simulink library "dspsigops"  (Simulink 8.2)
settings: Solver=ode45  SolverMode=SingleTasking  StartTime=0.0  StopTime=10.0  RelTol=1e-3
settings Model: RequirementInfo=9  ForwardingTableString=||__slOldName__||dspsigops/Zero Pad||__slNewName__||dspsigops/Pad||__slOldName__||dspsigops/Integer Delay||__slNewName__||dspobslib/Integer Delay  Creator=szlotkin  LastModifiedBy=mmclerno  CovMetricSettings=d  ExtModeAutoUpdateStatusClock=off

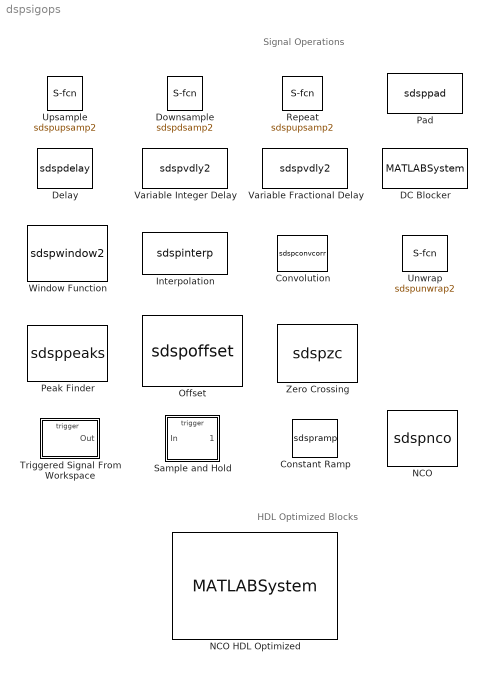
== system dspsigops ==
  note: Signal Operations
  note: HDL Optimized Blocks
  Constant Ramp : S-Function  FunctionName=sdspramp  Parameters=L, dim, Slope, Offset, isCustomFloat,isSigned,dTypeID,wordLength,fracBits,fracBitsMode  EnableBusSupport=off  mask(Constant Ramp){L=Rows, dim=1, Slope=1, Offset=0, additionalParams=off, allowOverrides=on, dataType=Same as input, isSigned=on, wordLen=16, udDataType=sfix(16), fracBitsMode=Best precision, numFracBits=15, OutDataTypeStr=Inherit: Same as input, LastOutDataTypeStr=Inherit: Same as input}
      mask prompts: L "Ramp length equals number of:"; dim "Dimension:"; additionalParams "------- Show additional parameters --------"; allowOverrides "Allow overrides from DSP Fixed-Point Attributes blocks"; dataType "Output data type:"; isSigned "Signed"; wordLen "Word length:"; udDataType "User-defined data type (e.g. sfix(16), float('single')):"; fracBitsMode "Set fraction length in output to:"; numFracBits "Fraction length:"; OutDataTypeStr "Output data type:"; LastOutDataTypeStr "Last output data type:"
      mask help:
      | Generate a ramp of length L, where L is the length of the input signal in the dimension specified by the 'Ramp length equals number of' parameter.
      |
      | The output of this block is calculated using output = [0:L-1] * slope + offset
      mask init:
      | blkh   = gcbh;
      | dtRows = dspblkGetConstantRampDTRowInfo();
      | outRow = dtRows{1};
      | if strcmpi(L, 'Elements in specified dimension')
      |     [dtInfo, dTypeID] = dspblkUDTMapperOutDType(blkh, outRow, 'dataType', (dim - 1));
      | else
      |     [dtInfo, dTypeID] = dspblkUDTMapperOutDType(blkh, outRow, 'dataType', 1);
      | end
      | isCustomFloat  = dtInfo.DataTypeIsCustomFloat;
      | if ~isCustomFloat
      |     isSigned   = dtInfo.DataTypeIsSigned;
      |     wordLength = dtInfo.DataTypeWordLength;
      |     fracBits   = dtInfo.DataTypeFracOrMantBits;
      | else
      |     isSigned   =  1; % nice default
      |     wordLength =  8; % nice default
      |     fracBits   =  0; % nice default
      | end
      mask Help: eval('blocksethelp');
      mask TypeOptions L: Rows | Columns | Elements in specified dimension
      mask Callback L: dspblkramp;
      mask TypeOptions dataType: Same as input | double | single | int8 | uint8 | int16 | uint16 | int32 | uint32 | boolean | Fixed-point | User-defined | Inherit via back propagation
      mask TypeOptions fracBitsMode: Best precision | User-defined
      mask Display: plot([.1 .9],[0 1]);
  Convolution : S-Function  DialogController=dspDDGCreate  DialogControllerArgs=DataTag0  FunctionName=sdspconvcorr  Parameters=domain,0,outputMin,outputMax,dtInfo.prodOutputMode,dtInfo.prodOutputWordLength,dtInfo.prodOutputFracLength,dtInfo.accumMode,dtInfo.accumWordLength,dtInfo.accumFracLength,dtInfo.outputMode,dtInfo.outputWordLength,dtInfo.outputFracLength,dtInfo.roundingMode,dtInfo.overflowMode  EnableBusSupport=off  mask(Convolution){domain=Time, additionalParams=off, allowOverrides=on, outputMode=Same as accumulator, outputWordLength=16, outputFracLength=15, outputDataTypeStr=Inherit: Same as accumulator, outputLastDataTypeStr=Inherit: Same as accumulator, outputMin=[], outputMax=[], accumMode=Inherit via internal rule, accumWordLength=32, accumFracLength=30, accumDataTypeStr=Inherit: Inherit via internal rule, accumLastDataTypeStr=Inherit: Inherit via internal rule, prodOutputMode=Inherit via internal rule, prodOutputWordLength=32, prodOutputFracLength=30, prodOutputDataTypeStr=Inherit: Inherit via internal rule, prodOutputLastDataTypeStr=Inherit: Inherit via internal rule, roundingMode=Floor, overflowMode=off, LockScale=off}
      mask prompts: domain "Computation domain:"; additionalParams "------- Show additional parameters -------"; allowOverrides "Allow overrides from DSP Fixed-Point Attributes blocks"; outputMode "Fixed-point output attributes:"; outputWordLength "Output word length:"; outputFracLength "Output fraction length:"; outputDataTypeStr "Output data type string:"; outputLastDataTypeStr "Last output data type string:"; outputMin "Output minimum:"; outputMax "Output maximum:"; accumMode "Fixed-point accumulator attributes:"; accumWordLength "Accumulator word length:"; accumFracLength "Accumulator fraction length:"; accumDataTypeStr "Accum data type string:"; accumLastDataTypeStr "Last accum data type string:"; prodOutputMode "Fixed-point product output attributes:"; prodOutputWordLength "Product output word length:"; prodOutputFracLength "Product output fraction length:"; prodOutputDataTypeStr "ProdOutput data type string:"; prodOutputLastDataTypeStr "Last prodOutput data type string:"; roundingMode "Round integer calculations toward:"; overflowMode "Saturate on integer overflow"; LockScale "Lock scaling"
      mask help: Convolve two inputs in the time or frequency domain. To allow the block to compute the convolution in the domain that minimizes the number of computations, set the 'Computation domain' parameter to 'Fastest'. To minimize memory usage, set the 'Computation domain' parameter to 'Time'.
      mask init:
      | blkh = gcbh;
      | dtRows = dspblkGetConvolutionDTRowInfo();
      | dtInfo = dspGetUDTFixptDataTypeInfo(blkh, dtRows, true);
      mask Help: eval('blocksethelp');
      mask TypeOptions domain: Time | Frequency | Fastest
      mask TypeOptions outputMode: Same as accumulator | Same as product output | Same as first input | Binary point scaling | Slope and bias scaling | User-defined
      mask TypeOptions accumMode: Inherit via internal rule | Same as product output | Same as first input | Binary point scaling | Slope and bias scaling | User-defined
      mask TypeOptions prodOutputMode: Inherit via internal rule | Same as first input | Binary point scaling | Slope and bias scaling | User-defined
      mask TypeOptions roundingMode: Ceiling | Convergent | Floor | Nearest | Round | Simplest | Zero
      mask Display: disp('CONV')
  DC Blocker : MATLABSystem  System=dsp.DCBlocker  Algorithm=IIR  NormalizedBandwidth=0.001  Length=8  Order=6
      mask Type: DCBlocker
      mask Display: disp('DC Blocker');
  Delay : S-Function  FunctionName=sdspdelay  Parameters=dly_unit, delay, dif_ic_for_ch, dif_ic_for_dly, ic, reset, InputProcessing  EnableBusSupport=off  mask(Delay){InputProcessing=Columns as channels (frame based), dly_unit=Samples, delay=1, ic_detail=off, dif_ic_for_ch=off, dif_ic_for_dly=off, ic=0, reset_popup=None}
      mask prompts: InputProcessing "Input processing:"; dly_unit "Delay units:"; delay "Delay (samples):"; ic_detail "--------------- Show additional parameters ---------------"; dif_ic_for_ch "Specify different initial conditions for each channel"; dif_ic_for_dly "Specify different initial conditions within a channel"; ic "Initial conditions:"; reset_popup "Reset port:"
      mask help: Delay the discrete-time input by a specified number of samples or frames.
      mask init:
      | dly_unitValue = get_param(gcbh, 'dly_unit');
      |  if (~iscell(ic)) 
      | 	ic = double(ic);
      |  end	
      | dspblkdelay('initInputProcessing', gcbh);
      | [str, ic] = dspblkdelay('init',dly_unitValue,double(delay), ic);
      | if (strcmp(str, 'Delay'))
      |     x1 = -10;
      |     y1 = -10;
      |     x2 = 0.35;
      |     y2 = 0.48;
      | else
      |     dx = min(0.35, 0.01*length(str));
      |     x1 = 0.42-dx;
      |     y1 = 0.4;
      |     x2 = 0.5-dx;
      |     y2 = 0.6;
      | end
      | reset = reset_popup-1;
      | if (reset == 0)
      | 	s.i1 = 1; s.i1s = '';
      | 	s.i2 = 1; s.i2s = '';
      | else
      | 	s.i1 = 1; s.i1s = 'In';
      | 	s.i2 = 2; s.i2s = 'Rst';
      | end
      mask Help: eval('blocksethelp');
      mask TypeOptions InputProcessing: Columns as channels (frame based) | Elements as channels (sample based) | Inherited (this choice will be removed - see release notes)
      mask Callback InputProcessing: dspblkdelay
      mask TypeOptions dly_unit: Samples | Frames
      mask Callback dly_unit: dspblkdelay
      mask TypeOptions reset_popup: None | Rising edge | Falling edge | Either edge | Non-zero sample
      mask Display:
      | text(x1, y1, 'z'); text(x2, y2, str);
      | port_label('input',s.i1,s.i1s);
      | port_label('input',s.i2,s.i2s);
  Downsample : S-Function  FunctionName=sdspdsamp2  Parameters=N,phase,ic,smode,fmode,InputProcessing,RateOptions  EnableBusSupport=off  mask(Downsample){N=2, phase=0, InputProcessing=Columns as channels (frame based), RateOptions=Enforce single-rate processing, smode=Allow multirate, fmode=Maintain input frame size, ic=0}
      mask prompts: N "Downsample factor, K:"; phase "Sample offset (0 to K-1):"; InputProcessing "Input processing:"; RateOptions "Rate options:"; smode "Sample-based mode:"; fmode "Frame-based mode:"; ic "Initial condition:"
      mask help: Downsample by an integer factor.
      mask init:
      | NValue = get_param(gcbh, 'N');
      | [s,x,y] = dspblkdsamp2('icon',N, NValue);
      | dspblkdsamp2('init', gcbh);
      mask Help: eval('blocksethelp');
      mask TypeOptions InputProcessing: Columns as channels (frame based) | Elements as channels (sample based) | Inherited (this choice will be removed - see release notes)
      mask Callback InputProcessing: dspblkdsamp2
      mask TypeOptions RateOptions: Enforce single-rate processing | Allow multirate processing
      mask Callback RateOptions: dspblkdsamp2
      mask TypeOptions smode: Allow multirate | Force single rate
      mask TypeOptions fmode: Maintain input frame size | Maintain input frame rate
      mask Display:
      | plot(x,y);
      | text(.6,.4,s);
  Interpolation : S-Function  FunctionName=sdspinterp  Parameters=InterpSource,InterpPoints,InterpMode,interpFilter,InvalidMode  EnableBusSupport=off  mask(Interpolation){InterpSource=Specify via dialog, InterpPoints=[1.1 4.8 2.67 1.6 3.2]', InterpMode=Linear, InterpL=3, InterpR=3, InterpAlpha=0.5, InvalidMode=Clip}
      mask prompts: InterpSource "Source of interpolation points:"; InterpPoints "Interpolation points:"; InterpMode "Interpolation mode:"; InterpL "Interpolation filter half-length:"; InterpR "Interpolation points per input sample:"; InterpAlpha "Normalized input bandwidth:"; InvalidMode "Out of range interpolation points:"
      mask help: Interpolate values between real-valued samples in one or more input vectors using linear or FIR interpolation.
      mask init:
      | ports = dspblkinterp('icon');
      | interpFilter = dspblkinterp('init', true, InterpR, InterpL, InterpAlpha);
      mask Help: eval('blocksethelp');
      mask TypeOptions InterpSource: Specify via dialog | Input port
      mask Callback InterpSource: dspblkinterp
      mask TypeOptions InterpMode: Linear | FIR
      mask Callback InterpMode: dspblkinterp
      mask TypeOptions InvalidMode: Clip | Clip and warn | Error
      mask Display:
      | disp('Interp')
      | port_label('input',ports.port1, ports.txt1);
      | port_label('input',ports.port2, ports.txt2);
      | port_label('output',ports.port3, ports.txt3);
  NCO : S-Function  DialogController=dspdialog.NCO  FunctionName=sdspnco  Parameters=AccIncSrc,AccInc,PhaseOffsetSrc,PhaseOffset,AccumWL,HasOutputPhaseError,HasDither,DitherWL,PNgeneratorLength,Formula,DataType,OutputWL,OutputFL,CompMethod,HasPhaseQuantizer,TableDepth,SampleTime,SamplesPerFrame  EnableBusSupport=off  mask(NCO){AccIncSrc=Input port, AccInc=100, PhaseOffsetSrc=Specify via dialog, PhaseOffset=0, AccumWL=16, HasDither=on, DitherWL=4, PNgeneratorLength=19, HasPhaseQuantizer=on, TableDepth=12, HasOutputPhaseError=off, Formula=Sine, DataType=Binary point scaling, OutputWL=16, OutputFL=14, CompMethod=Table lookup (no interpolation), SampleTime=1, SamplesPerFrame=1}
      mask prompts: AccIncSrc "Phase increment source:"; AccInc "Phase increment:"; PhaseOffsetSrc "Phase offset source:"; PhaseOffset "Phase offset:"; AccumWL "Phase accumulator size:"; HasDither "Add dither"; DitherWL "Number of dither bits:"; PNgeneratorLength "PN sequence generator length:"; HasPhaseQuantizer "Phase quantization"; TableDepth "Number of quantized bits:"; HasOutputPhaseError "Output phase quantization error"; Formula "Output signal:"; DataType "Output data type:"; OutputWL "Output word length:"; OutputFL "Output fraction length:"; CompMethod "Computation method:"; SampleTime "Output sample period (s):"; SamplesPerFrame "Samples per frame:"
      mask help: Generate a real or complex fixed-point sinusoidal signal.
      mask init:
      | str = dspblknco(AccIncSrc,PhaseOffsetSrc,Formula,HasOutputPhaseError,HasPhaseQuantizer);
      | set_param(gcbh, 'MaskDisplay', str);
      mask Help: eval('blocksethelp');
      mask TypeOptions AccIncSrc: Specify via dialog | Input port
      mask TypeOptions PhaseOffsetSrc: Specify via dialog | Input port
      mask TypeOptions Formula: Sine | Cosine | Complex exponential | Sine and cosine
      mask TypeOptions DataType: double | single | Binary point scaling
      mask TypeOptions CompMethod: Table lookup (no interpolation)
      mask Display: disp('NCO');port_label('input',1,'inc');port_label('output',1,'sin');
  NCO HDL Optimized : MATLABSystem  System=dsp.HDLNCO  PhaseIncrementSource=Input port  PhaseIncrement=100  PhaseOffsetSource=Property  PhaseOffset=0  DitherSource=Property  NumDitherBits=4  PhaseQuantization=on  NumQuantizerAccumulatorBits=12  LUTCompress=off  ResetAction=off  Waveform=Sine  PhasePort=off  AccumulatorWL=16  OutputDataType=Binary point scaling  OutputWL=16  OutputFL=14
      mask Type: dsp.HDLNCO
      mask Display:
      | disp(['NCO' char(10) 'HDL Optimized']);
      | port_label('input',1,'inc');
      | port_label('input',2,'validIn');
      | port_label('output',1,'sin');
      | port_label('output',2,'validOut');
  Offset : S-Function  FunctionName=sdspoffset  Parameters=mode,numDatOffPair,outWidthSpec,outWidth,actionOutRange  EnableBusSupport=off  mask(Offset){mode=Remove beginning samples, numDatOffPair=2, outWidthSpec=Same as input, outWidth=9, actionOutRange=Clip}
      mask prompts: numDatOffPair "Number of input data-offset pairs:"; outWidthSpec "Output port length:"; outWidth "Output length:"; actionOutRange "Action for out of range offset value:"
      mask help: Truncates input vectors by removing or keeping beginning or ending values. The resulting vectors are either truncated again or zero-padded to the specified output length.
      mask init:
      | dspblkoffset(numDatOffPair);
      mask Help: eval('blocksethelp');
      mask TypeOptions mode: Remove beginning samples | Remove ending samples | Keep beginning samples | Keep ending samples
      mask TypeOptions outWidthSpec: Same as input | User-defined
      mask Callback outWidthSpec: dspblkoffset;
      mask TypeOptions actionOutRange: Clip | Clip and warn | Error
      mask Display: port_label('input',1, 'In1'); port_label('output',1, 'Out1'); port_label('input',2, 'O1'); port_label('input',3, 'In2'); port_label('output',2, 'Out2'); port_label('input',4, 'O2'); disp('Offset');
  Pad : S-Function  FunctionName=sdsppad  Parameters=1,valSrc,padVal,spec,padNumOutColsSpecMethod,0,0,numOutCols,padNumOutRowsSpecMethod,0,0,numOutRows,trunc_flag,padAlong,padSigAt,outSizeMode,outSize,dimsToPad,padBeginning,padEnd,1  EnableBusSupport=off  mask(Pad){padAlong=Columns, dimsToPad=1, valSrc=Specify via dialog, padVal=0, spec=Output size, padNumOutRowsSpecMethod=User-specified, numOutRows=1, padNumOutColsSpecMethod=User-specified, numOutCols=1, isVarDimsMode=off, padBeginning=0, padEnd=0, outSizeMode=User-specified, outSize=1, padSigAt=End, trunc_flag=None, outputMode=Same as input, outputWordLength=0, outputFracLength=0, accumMode=Same as input, accumWordLength=0, accumFracLength=0, roundingMode=Floor, overflowMode=off, LockScale=off, truncOrWrapMode=Truncate, wrap_flag=None}
      mask prompts: padAlong "Pad over:"; dimsToPad "Dimensions to pad:"; valSrc "Pad value source:"; padVal "Pad value:"; spec "Specify:"; padNumOutRowsSpecMethod "Output column mode:"; numOutRows "Column size:"; padNumOutColsSpecMethod "Output row mode:"; numOutCols "Row size:"; isVarDimsMode "Variable dimension mode:"; padBeginning "Pad size at beginning:"; padEnd "Pad  size at end:"; outSizeMode "Output size mode:"; outSize "Output size:"; padSigAt "Pad signal at:"; trunc_flag "Action when truncation occurs:"; outputMode "Fixed-point output attributes:"; outputWordLength "Output word length"; outputFracLength "Output fraction length:"; accumMode "Fixed-point accumulator attributes:"; accumWordLength "Accumulator word length:"; accumFracLength "Accumulator fraction length:"; roundingMode "Round integer calculations toward:"; overflowMode "Saturate on integer overflow"; LockScale "Lock scaling"; truncOrWrapMode "Action when output size is smaller than input size:"; wrap_flag "Action when wrap occurs:"
      mask help: Append or prepend a constant value to the input along the specified dimensions. Truncation occurs when the specified output dimensions are shorter than the corresponding input dimensions.
      mask init:
      | ports = dspblkpad('icon');
      mask Help: eval('blocksethelp');
      mask TypeOptions padAlong: Columns | Rows | Columns and rows | None | Specified dimensions
      mask Callback padAlong: dspblkpad
      mask TypeOptions valSrc: Specify via dialog | Input port
      mask Callback valSrc: dspblkpad
      mask TypeOptions spec: Pad size | Output size
      mask Callback spec: dspblkpad
      mask TypeOptions padNumOutRowsSpecMethod: User-specified | Next power of two
      mask Callback padNumOutRowsSpecMethod: dspblkpad
      mask TypeOptions padNumOutColsSpecMethod: User-specified | Next power of two
      mask Callback padNumOutColsSpecMethod: dspblkpad
      mask TypeOptions outSizeMode: User-specified | Next power of two
      mask Callback outSizeMode: dspblkpad
      mask TypeOptions padSigAt: End | Beginning | Beginning and end
      mask TypeOptions trunc_flag: None | Warning | Error
      mask TypeOptions outputMode: Same as input | Binary point scaling | Slope and bias scaling
      mask TypeOptions accumMode: Same as input | Binary point scaling | Slope and bias scaling
      mask TypeOptions roundingMode: Floor | Nearest
      mask TypeOptions truncOrWrapMode: Truncate | Wrap
      mask TypeOptions wrap_flag: None | Warning | Error
      mask Display:
      | disp('Pad')
      | port_label('input',ports.port1, ports.txt1);
      | port_label('input',ports.port2, ports.txt2);
      | port_label('output',ports.port3, ports.txt3);
  Peak Finder : S-Function  DialogController=dspdialog.PeakFinder  DialogControllerArgs=DataTag3  FunctionName=sdsppeaks  Parameters=maxPeaks, polarity, NoiseDistinguish, thresh, outputIdx, outputVal, dtInfo.roundingMode, dtInfo.overflowMode  EnableBusSupport=off  mask(Peak Finder){polarity=Maxima and Minima, outputIdx=off, outputVal=off, maxPeaks=10, NoiseDistinguish=off, thresh=0, additionalParams=off, allowOverrides=off, roundingMode=Floor, overflowMode=off}
      mask prompts: polarity "Peak types:"; outputIdx "Output peak indices"; outputVal "Output peak values"; maxPeaks "Maximum number of peaks to find:"; NoiseDistinguish "Ignore peaks within threshold of neighboring values"; thresh "Threshold"; additionalParams "-------------- Show additional parameters ---------------"; allowOverrides "Allow overrides from DSP Fixed-Point Attributes blocks"; roundingMode "Round integer calculations toward:"; overflowMode "Saturate on integer overflow"
      mask help: Output the number of extrema (maxima and minima) in an input signal.
      mask init:
      | [s, dtInfo] = dspblkpeaks('icon',outputIdx,outputVal,polarity);
      mask Help: eval('blocksethelp');
      mask TypeOptions polarity: Maxima | Minima | Maxima and Minima
      mask TypeOptions roundingMode: Ceiling | Convergent | Floor | Nearest | Round | Simplest | Zero
      mask Display:
      | disp(['Find\n',s.txt]);
      | port_label('output',s.i1,s.s1);
      | port_label('output',s.i2,s.s2);
      | port_label('output',1,'Cnt');
      | port_label('output',s.i3,s.s3);
  Repeat : S-Function  FunctionName=sdspupsamp2  Parameters=N,0,ic,RateOptions,0,InputProcessing  EnableBusSupport=off  mask(Repeat){N=5, InputProcessing=Columns as channels (frame based), RateOptions=Enforce single-rate processing, ic=0, mode=Unused parameter value}
      mask prompts: N "Repetition count:"; InputProcessing "Input processing:"; RateOptions "Rate options:"; ic "Initial conditions:"; mode "Frame-based mode:"
      mask help: Repeat input samples N times.
      mask init:
      | NValue = get_param(gcbh, 'N');
      | s = dspblkrepeat2(gcbh,'icon',N, NValue);
      | dspblkrepeat2(gcbh,'init',mode);
      mask Help: eval('blocksethelp');
      mask TypeOptions InputProcessing: Columns as channels (frame based) | Elements as channels (sample based) | Inherited (this choice will be removed - see release notes)
      mask Callback InputProcessing: dspblkrepeat2
      mask TypeOptions RateOptions: Enforce single-rate processing | Allow multirate processing
      mask Callback RateOptions: dspblkrepeat2
      mask TypeOptions mode: Unused parameter value | Maintain input frame size | Maintain input frame rate
      mask Display: disp(s);
  Sample and Hold : Subsystem  TreatAsAtomicUnit=on  mask(Sample and Hold){trig=Rising edge, initCond=0, latchinput=off}
      mask prompts: trig "Trigger type:"; initCond "Initial condition:"; latchinput "Latch (buffer) input"
      mask help: Sample and hold the input signal. If Latch (buffer) input is selected, then this block produces the value of the input from the previous time step.
      mask init:
      | switch trig
      | case 1, s='rising';
      | case 2, s='falling';
      | case 3, s='either';
      | end
      | set_param([gcb '/Trigger'],'triggertype',s);
      | if (latchinput == 1)
      | 	set_param([gcb '/In'],'latchinput','on');
      | else
      | 	set_param([gcb '/In'],'latchinput','off');
      | end
      mask Help: eval('blocksethelp');
      mask TypeOptions trig: Rising edge | Falling edge | Either edge
      mask Display: disp('S/H')
  Triggered Signal From Workspace : Subsystem  TreatAsAtomicUnit=on  mask(Triggered Signal From Workspace){Signal=1:10, TriggerType=Falling edge, ic=0, SamplesPerFrame=1, OutputAfterFinalValue=Setting to zero}
      mask prompts: TriggerType "Trigger type:"; ic "Initial output:"; SamplesPerFrame "Samples per frame:"; OutputAfterFinalValue "Form output after final data value by:"
      mask help: Output successive signal samples obtained from the MATLAB workspace when a trigger event occurs. A signal matrix is interpreted as having one channel per column. Signal columns may be buffered into frames by specifying a number of samples per frame greater than 1. An M x N x P signal array outputs M x N matrices when a trigger event occurs. The samples per frame must be equal to 1 for 3 dimensional signal arrays.
      mask init:
      | SignalValue = get_param(gcbh, 'Signal');
      | s = dspblktsfw2('init', Signal,SamplesPerFrame);
      mask Help: eval('blocksethelp');
      mask TypeOptions TriggerType: Rising edge | Falling edge | Either edge
      mask TypeOptions OutputAfterFinalValue: Setting to zero | Holding final value | Cyclic repetition
      mask Display: disp(SignalValue);
  Unwrap : S-Function  FunctionName=sdspunwrap2  Parameters=tol, running, InputProcessing  EnableBusSupport=off  mask(Unwrap){tol=pi, InputProcessing=Columns as channels (frame based), running=off}
      mask prompts: tol "Tolerance (radians):"; InputProcessing "Input processing:"; running "Do not unwrap phase discontinuities between successive frames"
      mask help: Add or subtract multiples of 2pi to each input element to remove phase discontinuities (unwrap). The input units are radians.
      mask init:
      | dspblkunwrap(gcbh,'init');
      mask Help: eval('blocksethelp');
      mask TypeOptions InputProcessing: Columns as channels (frame based) | Elements as channels (sample based) | Inherited (this choice will be removed - see release notes)
      mask Callback InputProcessing: dspblkunwrap
      mask Display: plot(0,0,100,100,[16 16],[92 8],[8 92],[16 16],[16 48 48 80],[64 44 76 56],[64 64 58 64 70],[60 40 46 40 46],[69 82],[30 22],[],[],[52 65],[41 33])
  Upsample : S-Function  FunctionName=sdspupsamp2  Parameters=N,phase,ic,RateOptions,1,InputProcessing  EnableBusSupport=off  mask(Upsample){N=3, phase=0, InputProcessing=Columns as channels (frame based), RateOptions=Enforce single-rate processing, ic=0, mode=Unused parameter value}
      mask prompts: N "Upsample factor, L:"; phase "Sample offset (0 to L-1):"; InputProcessing "Input processing:"; RateOptions "Rate options:"; ic "Initial conditions:"; mode "Frame-based mode:"
      mask help: Upsample by inserting L-1 zeros between input samples.
      mask init:
      | NValue = get_param(gcbh, 'N');
      | [s,x,y] = dspblkupsamp2(gcbh,'icon',N,NValue);
      | dspblkupsamp2(gcbh,'init',mode);
      mask Help: eval('blocksethelp');
      mask TypeOptions InputProcessing: Columns as channels (frame based) | Elements as channels (sample based) | Inherited (this choice will be removed - see release notes)
      mask Callback InputProcessing: dspblkupsamp2
      mask TypeOptions RateOptions: Enforce single-rate processing | Allow multirate processing
      mask Callback RateOptions: dspblkupsamp2
      mask TypeOptions mode: Unused parameter value | Maintain input frame size | Maintain input frame rate
      mask Display:
      | plot(x,y)
      | text(.6,.4,s);
  Variable Fractional Delay : S-Function  DialogController=dspDDGCreate  DialogControllerArgs=DataTag8  FunctionName=sdspvdly2  Parameters=|  EnableBusSupport=off  mask(Variable Fractional Delay){mode=OBSOLETE, modeActive=Linear, dmax=100, InputProcessing=Columns as channels (frame based), L=4, FarrowL=4, R=10, alpha=1, ic=0, fallbackFIR=Clip to the minimum value necessary for centered kernel, fallbackFarrow=Clip to the minimum value necessary for centered kernel, noDFT=off, outputMode=Same as accumulator, outputWordLength=32, outputFracLength=10, prodOutputMode=Same as first input, prodOutputWordLength=32, prodOutputFracLength=10, accumMode=Same as product output, accumWordLength=32, accumFracLength=10, firstCoeffMode=Same word length as input, firstCoeffWordLength=32, firstCoeffFracLength=0, interProdMode=Same as first input, interProdWordLength=32, interProdFracLength=10, secondCoeffMode=Same as first input, secondCoeffWordLength=32, secondCoeffFracLength=10, memoryMode=Same as first input, memoryWordLength=32, memoryFracLength=10, roundingMode=Zero, overflowMode=off, LockScale=off}
      | modeActive,dmax,InputProcessing,b,ic, L,FarrowL, R, alpha, fallbackFIR, fallbackFarrow, noDFT,  dtInfo.firstCoeffMode ,
      | 
      | dtInfo.firstCoeffWordLength ,
      | 
      | dtInfo.firstCoeffFracLength ,
      | 
      | dtInfo.secondCoeffMode ,
      | 
      | dtInfo.secondCoeffWordLength,
      | 
      | dtInfo.secondCoeffFracLength ,
      | 
      | dtInfo.interProdMode ,
      | 
      | dtInfo.interProdWordLength ,
      | 
      | dtInfo.interProdFracLength ,
      | 
      | dtInfo.prodOutputMode ,
      | 
      | dtInfo.prodOutputWordLength ,
      | 
      | dtInfo.prodOutputFracLength ,
      | 
      | dtInfo.accumMode ,
      | 
      | dtInfo.accumWordLength ,
      | 
      | dtInfo.accumFracLength ,
      | 
      | dtInfo.memoryMode ,
      | 
      | dtInfo.memoryWordLength ,
      | 
      | dtInfo.memoryFracLength ,
      | 
      | dtInfo.outputMode, dtInfo.outputWordLength , dtInfo.outputFracLength ,
      | 
      | dtInfo.roundingMode ,
      | 
      | dtInfo.overflowMode
      mask prompts: mode "Mode Obsolete:"; modeActive "Interpolation structure:"; dmax "Maximum delay (samples):"; InputProcessing "Input processing:"; L "Interpolation filter half-length:"; FarrowL "Farrow filter length:"; R "Interpolation points per input sample:"; alpha "Normalized input bandwidth (0 to 1):"; ic "Initial conditions:"; fallbackFIR "Interpolation kernel selection mode:"; fallbackFarrow "Interpolation kernel selection mode:"; noDFT "Require an additional input delay value to disallow direct feedthrough"; outputMode "Fixed-point output attributes:"; outputWordLength "Output word length:"; outputFracLength "Output fraction length:"; prodOutputMode "Fixed-point product output attributes:"; prodOutputWordLength "Product output word length:"; prodOutputFracLength "Product output fraction length:"; accumMode "Fixed-point accumulator attributes:"; accumWordLength "Accumulator word length:"; accumFracLength "Accumulator fraction length:"; firstCoeffMode "Fixed-point coefficients attributes:"; firstCoeffWordLength "Coefficients word length:"; firstCoeffFracLength "Coefficients word length:"; interProdMode "Fixed-point product 2 output attributes:"; interProdWordLength "Product output word length:"; interProdFracLength "Product output fraction length:"; secondCoeffMode "Fixed-point accumulator 2 attributes:"; secondCoeffWordLength "Accumulator 2 word length:"; secondCoeffFracLength "Accumulator 2 fraction length:"; memoryMode "Fixed-point multiplicand attributes:"; memoryWordLength "Multiplicand word length:"; memoryFracLength "Multiplicand fraction length:"; roundingMode "Round integer calculations toward:"; overflowMode "Saturate on integer overflow"; LockScale "Lock scaling"
      mask help:
      | Delay discrete-time input by the time-varying fractional number of sample periods specified by the 'Delay' input. The block provides Linear, FIR, and Farrow interpolation modes. In FIR mode, the filter is designed using the 'intfilt' function from the Signal Processing Toolbox.
      |
      | The input delay is clipped to a valid range (Dmin to Dmax) that is determined by the parameter settings.
      mask init:
      | blkh = gcbh;
      | dtInfo = dspGetFixptDataTypeInfo(blkh,383);
      | if (modeActive == 3)
      |     [b] = dspblkvfdly2(blkh,modeActive,FarrowL);
      | else
      |     [b] = dspblkvfdly2(blkh,modeActive,R,L,alpha);
      | end
      mask Help: eval('blocksethelp');
      mask TypeOptions mode: Linear interpolation | FIR interpolation | OBSOLETE
      mask TypeOptions modeActive: Linear | FIR | Farrow
      mask TypeOptions InputProcessing: Columns as channels (frame based) | Elements as channels (sample based) | Inherited (this choice will be removed - see release notes)
      mask TypeOptions fallbackFIR: Clip to the minimum value necessary for centered kernel | Switch to linear interpolation if kernel cannot be centered
      mask TypeOptions fallbackFarrow: Clip to the minimum value necessary for centered kernel | Use off-centered kernel
      mask TypeOptions outputMode: Same as accumulator | Same as first input | Binary point scaling | Slope and bias scaling
      mask TypeOptions prodOutputMode: Same as first input | Binary point scaling | Slope and bias scaling
      mask TypeOptions accumMode: Same as product output | Same as first input | Binary point scaling | Slope and bias scaling
      mask TypeOptions firstCoeffMode: Same word length as input | Specify word length
      mask TypeOptions interProdMode: Same as first input | Binary point scaling | Slope and bias scaling
      mask TypeOptions secondCoeffMode: Same as first input | Binary point scaling | Slope and bias scaling
      mask TypeOptions memoryMode: Same as first input | Binary point scaling | Slope and bias scaling
      mask TypeOptions roundingMode: Ceiling | Convergent | Floor | Nearest | Round | Simplest | Zero
      mask Display:
      | text(0.5,0.4,'z','horiz','right')
      | text(0.5,0.6,'-f','horiz','left')
      | port_label('input',1,'In')
      | port_label('input',2,'Delay')
  Variable Integer Delay : S-Function  FunctionName=sdspvdly2  Parameters=0,dmax,InputProcessing,0,ic,0,0,0,0,0,0,noDFT,2,2,2,2,2,2,2,2,2,2,2,2,2,2,2,2,2,2,2,2,2,2,2  EnableBusSupport=off  mask(Variable Integer Delay){dmax=100, InputProcessing=Columns as channels (frame based), ic=0, noDFT=off}
      mask prompts: dmax "Maximum delay (samples):"; InputProcessing "Input processing:"; ic "Initial conditions:"; noDFT "Disable direct feedthrough by increasing minimum possible delay by one"
      mask help: Delay discrete-time input by a time-varying integer number of sample periods specified by the "delay" input.
      mask init:
      | dspSetFrameUpgradeParameter(gcbh, 'InputProcessing','Inherited (this choice will be removed - see release notes)');
      mask Help: eval('blocksethelp');
      mask TypeOptions InputProcessing: Columns as channels (frame based) | Elements as channels (sample based) | Inherited (this choice will be removed - see release notes)
      mask Display:
      | text(0.5,0.4,'z','horiz','right')
      | text(0.5,0.6,'-i','horiz','left')
      | port_label('input',1,'In')
      | port_label('input',2,'Delay')
      | port_label('output',1,'Out')
  Window Function : S-Function  DialogController=dspDDGCreate  DialogControllerArgs=DataTag10  FunctionName=sdspwindow2  Parameters=winmode,N,sampmode,samptime,wintype,winsamp,Rs,beta,numSidelobes,sidelobeLevel,UserWindow,OptParams,UserParams,RowConvenienceOn,dtInfo.DataTypeIsCustomFloat,dtInfo.DataTypeIsSigned,dTypeID,dtInfo.DataTypeWordLength,dtInfo.DataTypeFracOrMantBits,fixptInfo.firstCoeffMode,fixptInfo.firstCoeffWordLength,fixptInfo.firstCoeffFracLength,fixptInfo.prodOutputMode,fixptInfo.prodOutputWordLength,fixptInfo.prodOutputFracLength,fixptInfo.outputMode,fixptInfo.outputWordLength,fixptInfo.outputFracLength,fixptInfo.roundingMode,fixptInfo.overflowMode  EnableBusSupport=off  mask(Window Function){winmode=Apply window to input, wintype=Hamming, sampmode=Continuous, samptime=1, N=64, Rs=50, beta=10, winsamp=Symmetric, UserWindow=hamming, OptParams=off, UserParams={'symmetric'}, RowConvenienceOn=on, additionalParams=off, allowOverrides=on, dataType=double, isSigned=on, wordLen=16, udDataType=sfix(16), fracBitsMode=Best precision, numFracBits=15, firstCoeffMode=Same word length as input, firstCoeffWordLength=16, firstCoeffFracLength=15, prodOutputMode=Inherit via internal rule, prodOutputWordLength=16, prodOutputFracLength=15, outputMode=Same as product output, outputWordLength=16, outputFracLength=15, roundingMode=Floor, overflowMode=off, LockScale=off, numSidelobes=4, sidelobeLevel=-30}
      mask prompts: winmode "Operation:"; wintype "Window type:"; sampmode "Sample mode:"; samptime "Sample time:"; N "Window length:"; Rs "Stopband attenuation in dB:"; winsamp "Sampling:"; UserWindow "Window function name:"; OptParams "Additional parameters for user defined window"; UserParams "Window function parameters:"; RowConvenienceOn "Perform row convenience"; additionalParams "------- Show additional parameters --------"; allowOverrides "Allow overrides from DSP Fixed-Point Attributes blocks"; dataType "Output data type:"; isSigned "Signed"; wordLen "Word length:"; udDataType "User-defined data type  (e.g. sfix(16), float('single')):"; fracBitsMode "Set fraction length in output to:"; numFracBits "Fraction length:"; firstCoeffMode "Fixed-point window attributes:"; firstCoeffWordLength "Window word length:"; firstCoeffFracLength "Window fraction length:"; prodOutputMode "Fixed-point product output attributes:"; prodOutputWordLength "Product output word length:"; prodOutputFracLength "Product output fraction length:"; outputMode "Fixed-point output attributes:"; outputWordLength "Output word length:"; outputFracLength "Output fraction length:"; roundingMode "Round integer calculations towards:"; overflowMode "Saturate on integer overflow"; LockScale "Lock scaling"; numSidelobes "Number of sidelobes:"; sidelobeLevel "Sidelobe level (db):"
      mask help: Generate a window function and/or apply a window function to an input signal.
      mask init:
      | [x,y,str,ports,w,dtInfo,dTypeID,fixptInfo]=dspblkwinfcn2('init');
      mask Help: eval('blocksethelp');
      mask TypeOptions winmode: Apply window to input | Generate window | Generate and apply window
      mask TypeOptions wintype: Bartlett | Blackman | Boxcar | Chebyshev | Hamming | Hann | Hanning | Kaiser | Taylor | Triang | User defined
      mask TypeOptions sampmode: Discrete | Continuous
      mask TypeOptions winsamp: Symmetric | Periodic
      mask TypeOptions dataType: double | single | Fixed-point | User-defined | Inherit via back propagation
      mask TypeOptions fracBitsMode: Best precision | User-defined
      mask TypeOptions firstCoeffMode: Same word length as input | Specify word length | Binary point scaling | Slope and bias scaling | User-defined
      mask TypeOptions prodOutputMode: Inherit via internal rule | Same as input | Binary point scaling | Slope and bias scaling | User-defined
      mask TypeOptions outputMode: Same as product output | Same as input | Binary point scaling | Slope and bias scaling | User-defined
      mask TypeOptions roundingMode: Ceiling | Convergent | Floor | Nearest | Round | Simplest | Zero
      mask Display:
      | plot(x,y); text(.2,.85,str);
      | port_label(ports(1).type,ports(1).port,ports(1).txt);
      | port_label(ports(2).type,ports(2).port,ports(2).txt);
      | port_label(ports(3).type,ports(3).port,ports(3).txt);
  Zero Crossing : S-Function  FunctionName=sdspzc  Parameters=InputProcessing,1,1  EnableBusSupport=off  mask(Zero Crossing){InputProcessing=Columns as channels (frame based)}
      mask prompts: InputProcessing "Input processing:"
      mask help: Counts the number of zero crossings in a signal.
      mask init:
      | dspSetFrameUpgradeParameter(gcbh, 'InputProcessing','Inherited (this choice will be removed - see release notes)');
      mask Help: eval('blocksethelp');
      mask TypeOptions InputProcessing: Columns as channels (frame based) | Elements as channels (sample based) | Inherited (this choice will be removed - see release notes)
      mask Display:
      | disp(['Zero\nCrossing']);
      | port_label('output',1,'Cnt');

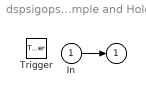
== system dspsigops/Sample and Hold ==
  In : Inport
  Trigger : TriggerPort  ZeroCross=off
  " " : Outport  InitialOutput=initCond
  wires:
  In/1 -> " "/1

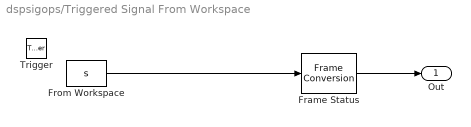
== system dspsigops/Triggered Signal From Workspace ==
  Trigger : TriggerPort  TriggerType=falling  StatesWhenEnabling=reset  ZeroCross=off
  Frame Status : FrameConversion  OutFrame=Sample-based
  From Workspace : FromWorkspace  VariableName=s  Interpolate=off  OutputAfterFinalValue=Setting to zero
  Out : Outport  InitialOutput=ic
  wires:
  From Workspace/1 -> Frame Status/1
  Frame Status/1 -> Out/1
